simulink model "UpravljanjeNelinearni"  (R2018a)
settings: Solver=VariableStepAuto  StartTime=0.0  StopTime=9  RelTol=1e-3  EnableMultiTasking=on
values from neighbouring files (symbols this model uses):
  Bv = 1.349*10^(-5)    (= 1.349e-05)    [Podaci.m]    (also in Podaci.mat)
  F0 = 0.1717    [Podaci.m]    (also in Podaci.mat)
  idn = Odgovor(2)    [nominale.m]
  iqn = Odgovor(3)    [nominale.m]
  J0 = 3.26*10^-3    (= 0.00326)    [Podaci.m]    (also in Podaci.mat)
  Ls = Ld    (= 0.03682)    [Podaci.m]    (also in Podaci.mat)
  m = 3    [Podaci.m]    (also in Podaci.mat)
  mhn = 0.3    [nominale.m]
  np = 2    [Podaci.m]    (also in Podaci.mat)
  Rs = 16.7    [Podaci.m]    (also in Podaci.mat)
  wmn = nn*pi/30    (= 314.159265359)    [nominale.m]
settings Model: Creator=Bane  LastModifiedBy=lakim
settings DataIOCC: LimitDataPoints=on
settings OptimizationCC: LifeSpan=inf
settings DebuggingCC: AllowSymbolicDim=off  SFUnexpectedBacktrackingDiag=warning  SFNoUnconditionalDefaultTransitionDiag=warning  SFExecutionAtInitializationDiag=none
settings ModelReferenceCC: PropagateSignalLabelsOutOfModel=off
settings CodeAppCC: StateflowObjectComments=on
settings GRTTargetCC: TargetLangStandard=C89/C90 (ANSI)
settings ConfigComp: CovMetricSettings=dw  CovHtmlReporting=on  CovSaveCumulativeToWorkspaceVar=on  CovSaveSingleToWorkspaceVar=on  CovExternalEMLEnable=off

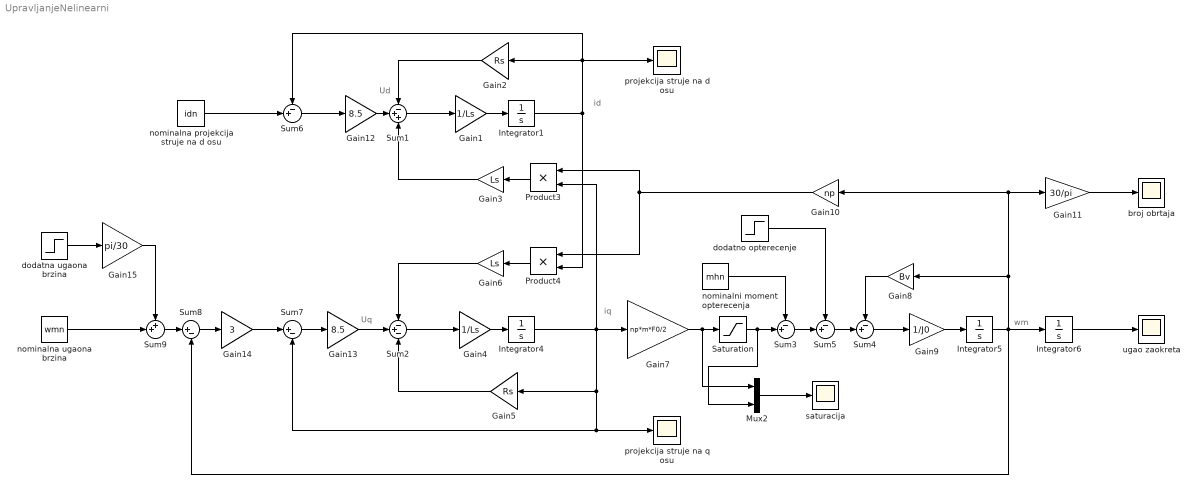
== system UpravljanjeNelinearni ==
  note: Uq
  note: iq
  note: id
  note: Ud
  note: wm
  Gain1 : Gain  Gain=1/Ls
  Gain10 : Gain  Gain=np
  Gain11 : Gain  Gain=30/pi
  Gain12 : Gain  Gain=8.5
  Gain13 : Gain  Gain=8.5
  Gain14 : Gain  Gain=3
  Gain15 : Gain  Gain=pi/30
  Gain2 : Gain  Gain=Rs
  Gain3 : Gain  Gain=Ls
  Gain4 : Gain  Gain=1/Ls
  Gain5 : Gain  Gain=Rs
  Gain6 : Gain  Gain=Ls
  Gain7 : Gain  Gain=np*m*F0/2
  Gain8 : Gain  Gain=Bv
  Gain9 : Gain  Gain=1/J0
  Integrator1 : Integrator  InitialCondition=idn
  Integrator4 : Integrator  InitialCondition=iqn
  Integrator5 : Integrator  InitialCondition=wmn
  Integrator6 : Integrator
  Mux2 : Mux  Inputs=2
  Product3 : Product
  Product4 : Product
  Saturation : Saturate  UpperLimit=8  LowerLimit=-8
  Sum1 : Sum  Inputs=-++
  Sum2 : Sum  Inputs=-+-
  Sum{3..6} (4 alike) : Sum  Inputs=-+|
  Sum7 : Sum  Inputs=|+-
  Sum8 : Sum  Inputs=|+-
  Sum9 : Sum  Inputs=++|
  "broj obrtaja " : Scope
  dodatna ugaona brzina : Step  Time=3  After=100  SampleTime=0
  dodatno opterecenje : Step  Time=6  SampleTime=0
  nominalna projekcija struje na d osu : Constant  Value=idn
  nominalna ugaona brzina : Constant  Value=wmn
  nominalni moment opterecenja : Constant  Value=mhn
  projekcija struje na q osu : Scope
  projekcija struje na d osu : Scope
  saturacija : Scope
  ugao zaokreta : Scope
  wires:
  Gain1/1 -> Integrator1/1
  Gain2/1 -> Sum1/1
  Sum1/1 -> Gain1/1
  Gain12/1 -> Sum1/2
  Product3/1 -> Gain3/1
  Gain3/1 -> Sum1/3
  Gain4/1 -> Integrator4/1
  Sum2/1 -> Gain4/1
  Gain13/1 -> Sum2/2
  Product4/1 -> Gain6/1
  Gain6/1 -> Sum2/1
  Gain5/1 -> Sum2/3
  Gain9/1 -> Integrator5/1
  Integrator5/1 -> Sum8/2, Integrator6/1, Gain11/1, Gain10/1, Gain8/1
  nominalni moment opterecenja/1 -> Sum3/1
  Sum4/1 -> Gain9/1
  Gain8/1 -> Sum4/1
  Gain10/1 -> Product4/1, Product3/1
  Gain11/1 -> "broj obrtaja "/1
  Integrator6/1 -> ugao zaokreta/1
  Sum3/1 -> Sum5/2
  Sum5/1 -> Sum4/2
  dodatno opterecenje/1 -> Sum5/1
  Sum6/1 -> Gain12/1
  Sum7/1 -> Gain13/1
  Sum8/1 -> Gain14/1
  nominalna ugaona brzina/1 -> Sum9/2
  Sum9/1 -> Sum8/1
  Gain15/1 -> Sum9/1
  dodatna ugaona brzina/1 -> Gain15/1
  Saturation/1 -> Mux2/2, Sum3/2
  Gain7/1 -> Mux2/1, Saturation/1
  Gain14/1 -> Sum7/1
  Mux2/1 -> saturacija/1
  Integrator1/1 -> Product4/2, Sum6/1, Gain2/1, projekcija struje na d osu/1
  Integrator4/1 -> Product3/2, Gain7/1, Sum7/2, projekcija struje na q osu/1, Gain5/1
  nominalna projekcija struje na d osu/1 -> Sum6/2
